simulink model "Solar_PV_IV_PV_Characteristics"  (R2024b)
settings: Solver=VariableStepAuto  StartTime=0.0  StopTime=4  RelTol=1e-3
values from neighbouring files (symbols this model uses):
  Ego = 1.1    [Soalr_Modeling_Parameters.m]
  Isc = 7.95    [Soalr_Modeling_Parameters.m]
  k = 1.380648e-23    [Soalr_Modeling_Parameters.m]
  ki = 0.0032    [Soalr_Modeling_Parameters.m]
  n = 1.29    [Soalr_Modeling_Parameters.m]
  Ns = 60    [Soalr_Modeling_Parameters.m]
  q = 1.602e-19    [Soalr_Modeling_Parameters.m]
  Rs = 0.1896    [Soalr_Modeling_Parameters.m]
  Rsh = 106.18    [Soalr_Modeling_Parameters.m]
  Tn = 298    [Soalr_Modeling_Parameters.m]
  Voc = 36.06    [Soalr_Modeling_Parameters.m]
libraries: simulink x1
settings Model: Creator=MULUK  LastModifiedBy=MULUK

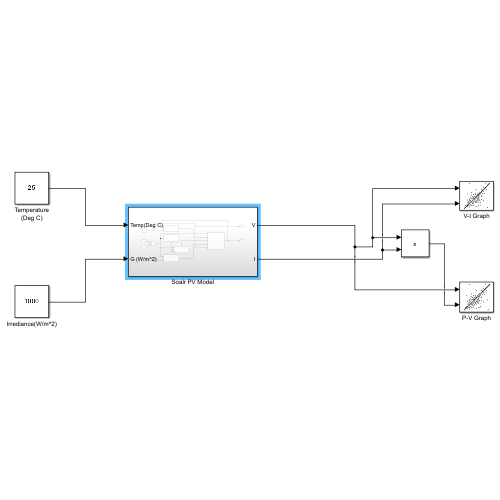
[thumbnail: Simulink's stored preview of the top-level diagram]
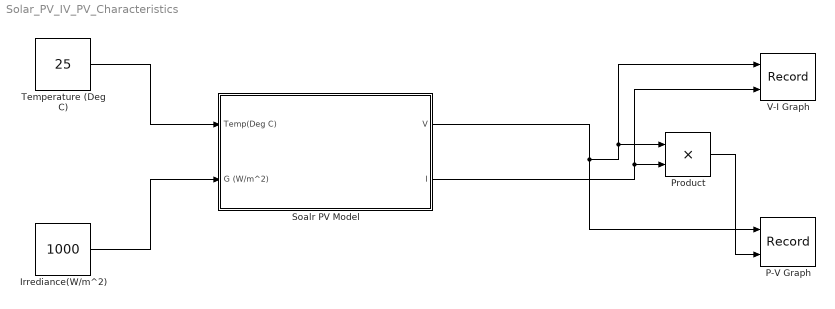
== system Solar_PV_IV_PV_Characteristics ==
  Irrediance(W/m^2) : Constant  Value=1000
  P-V Graph : Record  FileSettingsInternal="{\"entries\":[{\"content\":{\"excelSettings\":{\"content\":{},\"type\":\"Streamout.ExcelSettings\"}},\"type\":\"Streamout.FileSettingStorage\",\"uuid\":\"\"}],\"packageUris\":[\"http:\\/\\/schema.mathworks.com\\/mf0\\/streamout_blocks\\/R2020a\"],\"version\":\"1.0\"}"  Layout=[1 1]  SignalsInternal="{\"entries\":[{\"content\":{\"signals\":[{\"content\":{\"blockPath\":[],\"dimensions\":[1],\"domain\":\"\",\"lineColor\":\"#a2142f\",\"plots\":[ 1 ],\"port\":1,\"sid\":[\"\"],\"signalID\":1,\"signalName\":\"Soalr PV Model:1\"},\"type\":\"RecordBlkView.Signal\",\"uuid\":\"\"},{\"content\":{\"blockPath\":[],\"dimensions\":[1],\"domain\":\"\",\"lineColor\":\"#139fff\",\"plots\":[ 1 ],\"port\":2,\"sid\":[\"\"],\"signalID\":2,\"signalName\":\"Product\"},\"type\":\"RecordBlkView.Signal\",\"uuid\":\"\"}]},\"type\":\"RecordBlkView.InputSignals\",\"uuid\":\"\"}],\"packageUris\":[\"http:\\/\\/schema.mathworks.com\\/mf0\\/streamout_blocks\\/R2020a\"],\"version\":\"1.0\"}"  VisualizationBindings="{\"xyplotplugin\":{\"info\":[{\"series\":[{\"bindingParametersList\":[{\"parameter\":\"X-Axis\",\"signalID\":1,\"signalName\":\"Soalr PV Model:1\"},{\"parameter\":\"Y-Axis\",\"signalID\":2,\"signalName\":\"Product\"}],\"seriesID\":0}],\"subplotID\":1}]}}"  CompatibilityTag=XY
  Product : Product
  Soalr PV Model : Subsystem
  Temperature (Deg C) : Constant  Value=25
  V-I Graph : Record  FileSettingsInternal="{\"entries\":[{\"content\":{\"excelSettings\":{\"content\":{},\"type\":\"Streamout.ExcelSettings\"}},\"type\":\"Streamout.FileSettingStorage\",\"uuid\":\"\"}],\"packageUris\":[\"http:\\/\\/schema.mathworks.com\\/mf0\\/streamout_blocks\\/R2020a\"],\"version\":\"1.0\"}"  Layout=[1 1]  SignalsInternal="{\"entries\":[{\"content\":{\"signals\":[{\"content\":{\"blockPath\":[],\"dimensions\":[1],\"domain\":\"\",\"lineColor\":\"#a2142f\",\"plots\":[ 1 ],\"port\":1,\"sid\":[\"\"],\"signalID\":1,\"signalName\":\"Soalr PV Model:1\"},\"type\":\"RecordBlkView.Signal\",\"uuid\":\"\"},{\"content\":{\"blockPath\":[],\"dimensions\":[1],\"domain\":\"\",\"lineColor\":\"#139fff\",\"plots\":[ 1 ],\"port\":2,\"sid\":[\"\"],\"signalID\":2,\"signalName\":\"Soalr PV Model:2\"},\"type\":\"RecordBlkView.Signal\",\"uuid\":\"\"}]},\"type\":\"RecordBlkView.InputSignals\",\"uuid\":\"\"}],\"packageUris\":[\"http:\\/\\/schema.mathworks.com\\/mf0\\/streamout_blocks\\/R2020a\"],\"version\":\"1.0\"}"  VisualizationBindings="{\"xyplotplugin\":{\"info\":[{\"series\":[{\"bindingParametersList\":[{\"parameter\":\"X-Axis\",\"signalID\":1,\"signalName\":\"Soalr PV Model:1\"},{\"parameter\":\"Y-Axis\",\"signalID\":2,\"signalName\":\"Soalr PV Model:2\"}],\"seriesID\":0}],\"subplotID\":1}]}}"  CompatibilityTag=XY
  wires:
  Temperature (Deg C)/1 -> Soalr PV Model/1(Temp(Deg C))
  Irrediance(W/m^2)/1 -> Soalr PV Model/2(G (W/m^2))
  Soalr PV Model/1(V) -> P-V Graph/1, Product/1, V-I Graph/1
  Soalr PV Model/2(I) -> V-I Graph/2, Product/2
  Product/1 -> P-V Graph/2

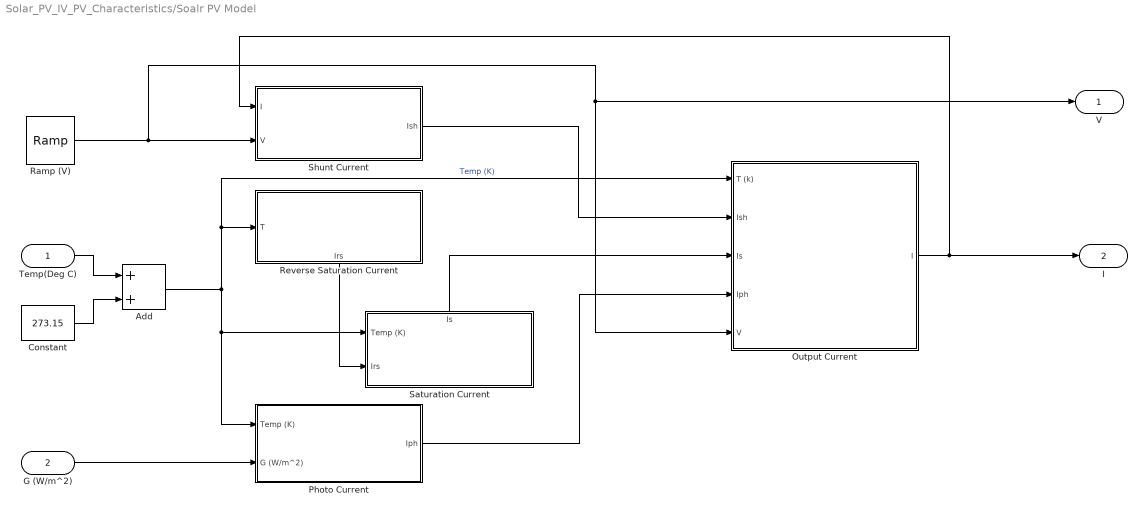
== system Solar_PV_IV_PV_Characteristics/Soalr PV Model ==
  Temp(Deg C) : Inport
  G (W/m^2) : Inport  Port=2
  " Saturation Current" : Subsystem
      settings: PortSchema="{\"entries\":[{\"content\":{\"sides\":[{\"content\":{\"connectorIds\":[\"In1\",\"In2\"]},\"type\":\"ConnectorPlacement.EquallySpacedRectSide\",\"uuid\":\"228251db-ac4b-41cf-ba5c-a510b5a8f8e4\"},{\"content\":{\"side\":\"RIGHT\"},\"type\":\"ConnectorPlacement.EquallySpacedRectSide\",\"uuid\":\"dc30eacc-74c4-4b6b-93d0-5a4bc4de7db7\"},{\"content\":{\"connectorIds\":[\"Out1\"],\"side\":\"TOP\"},\"type\":\"ConnectorPlacement.EquallySpacedRectSide\",\"uuid\":\"0f21fec9-16ef-4863-8682-a91fb4282025\"}]},\"type\":\"ConnectorPlacement.EquallySpacedConnector\",\"uuid\":\"707e5a0b-264d-4615-9fee-634224bb9e7b\"}],\"packageUris\":[\"http://schema.mathworks.com/mf0/Connector/R2020b\"],\"version\":\"1.0\"}"
  Add : Sum
  Constant : Constant  Value=273.15
  Output Current : Subsystem
  Photo Current : Subsystem
  Ramp (V) : simulink/Sources/Ramp  slope=10  start=0  InitialOutput=0
  Reverse Saturation Current : Subsystem
      settings: PortSchema="{\"entries\":[{\"content\":{\"sides\":[{\"content\":{\"connectorIds\":[\"In1\"]},\"type\":\"ConnectorPlacement.EquallySpacedRectSide\",\"uuid\":\"15512ed6-b5a7-405b-8341-08cd34b41276\"},{\"content\":{\"side\":\"RIGHT\"},\"type\":\"ConnectorPlacement.EquallySpacedRectSide\",\"uuid\":\"2cf76314-964e-48ba-8c80-893730139cda\"},{\"content\":{\"side\":\"TOP\"},\"type\":\"ConnectorPlacement.EquallySpacedRectSide\",\"uuid\":\"5ff35256-eb4a-4971-9008-324c8c50e0f9\"},{\"content\":{\"connectorIds\":[\"Out1\"],\"side\":\"BOTTOM\"},\"type\":\"ConnectorPlacement.EquallySpacedRectSide\",\"uuid\":\"1ee23ac2-1bc7-4858-ab4d-5fdcca5de137\"}]},\"type\":\"ConnectorPlacement.EquallySpacedConnector\",\"uuid\":\"a755481f-b56d-49f1-ba2a-78615b253991\"}],\"packageUris\":[\"http://schema.mathworks.com/mf0/Connector/R2020b\"],\"version\":\"1.0\"}"
  "Shunt Current " : Subsystem
  V : Outport
  I : Outport  Port=2
  wires:
  Temp(Deg C)/1 -> Add/1
  Constant/1 -> Add/2
  Add/1 -> Output Current/1(T (k)), Reverse Saturation Current/1(T), Photo Current/1(Temp (K)), " Saturation Current"/1(Temp (K))  "Temp (K)"
  G (W/m^2)/1 -> Photo Current/2(G (W/m^2))
  Reverse Saturation Current/1(Irs) -> " Saturation Current"/2(Irs)
  "Shunt Current "/1(Ish) -> Output Current/2(Ish)
  Photo Current/1(Iph) -> Output Current/4(Iph)
  " Saturation Current"/1(Is) -> Output Current/3(Is)
  Output Current/1(I) -> I/1, "Shunt Current "/1(I)
  Ramp (V)/1 -> V/1, Output Current/5(V), "Shunt Current "/2(V)

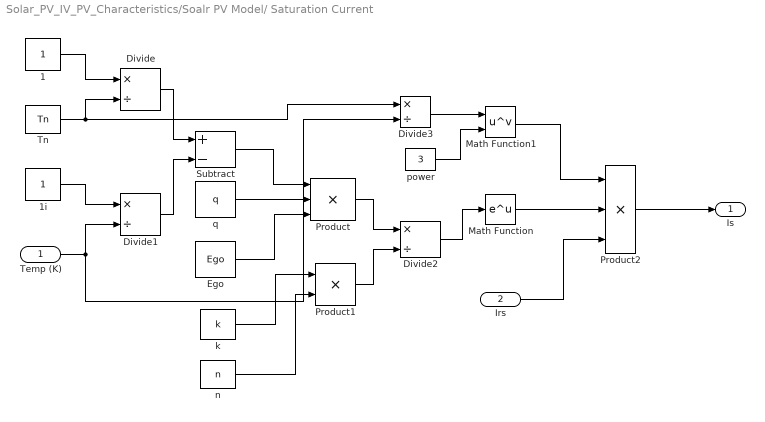
== system Solar_PV_IV_PV_Characteristics/Soalr PV Model/ Saturation Current ==
  Temp (K) : Inport
  Irs : Inport  Port=2
  1 : Constant
  1i : Constant
  Divide{,1..3} (4 alike) : Product  Inputs=*/
  Ego : Constant  Value=Ego
  Math Function : Math
  Math Function1 : Math  Operator=pow
  Product : Product  Inputs=3
  Product1 : Product
  Product2 : Product  Inputs=3
  Subtract : Sum  Inputs=+-
  Tn : Constant  Value=Tn
  k : Constant  Value=k
  n : Constant  Value=n
  power : Constant  Value=3
  q : Constant  Value=q
  Is : Outport
  wires:
  1/1 -> Divide/1
  Tn/1 -> Divide/2, Divide3/1
  1i/1 -> Divide1/1
  Temp (K)/1 -> Divide1/2, Divide3/2
  Divide/1 -> Subtract/1
  Divide1/1 -> Subtract/2
  Subtract/1 -> Product/1
  q/1 -> Product/2
  Ego/1 -> Product/3
  k/1 -> Product1/1
  n/1 -> Product1/2
  Product/1 -> Divide2/1
  Product1/1 -> Divide2/2
  Divide2/1 -> Math Function/1
  Divide3/1 -> Math Function1/1
  power/1 -> Math Function1/2
  Math Function/1 -> Product2/2
  Math Function1/1 -> Product2/1
  Irs/1 -> Product2/3
  Product2/1 -> Is/1

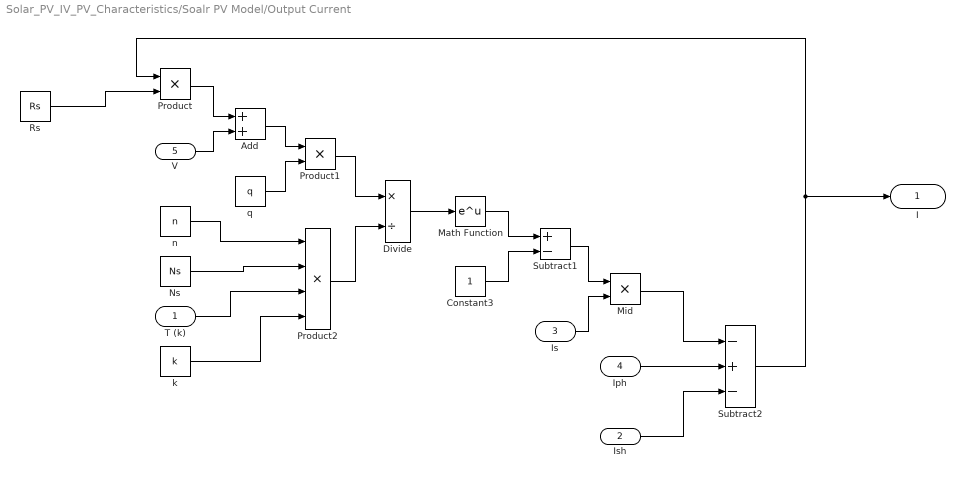
== system Solar_PV_IV_PV_Characteristics/Soalr PV Model/Output Current ==
  T (k) : Inport
  Ish : Inport  Port=2
  Is : Inport  Port=3
  Iph : Inport  Port=4
  V : Inport  Port=5
  Add : Sum
  Constant3 : Constant
  Divide : Product  Inputs=*/
  Math Function : Math
  Mid : Product
  Ns : Constant  Value=Ns
  Product : Product
  Product1 : Product
  Product2 : Product  Inputs=4
  Rs : Constant  Value=Rs
  Subtract1 : Sum  Inputs=+-
  Subtract2 : Sum  Inputs=-+-
  k : Constant  Value=k
  n : Constant  Value=n
  q : Constant  Value=q
  I : Outport
  wires:
  Subtract2/1 -> Product/1, I/1
  Rs/1 -> Product/2
  Product/1 -> Add/1
  V/1 -> Add/2
  q/1 -> Product1/2
  Add/1 -> Product1/1
  n/1 -> Product2/1
  T (k)/1 -> Product2/3
  k/1 -> Product2/4
  Ns/1 -> Product2/2
  Product1/1 -> Divide/1
  Product2/1 -> Divide/2
  Divide/1 -> Math Function/1
  Math Function/1 -> Subtract1/1
  Constant3/1 -> Subtract1/2
  Subtract1/1 -> Mid/1
  Is/1 -> Mid/2
  Mid/1 -> Subtract2/1
  Iph/1 -> Subtract2/2
  Ish/1 -> Subtract2/3

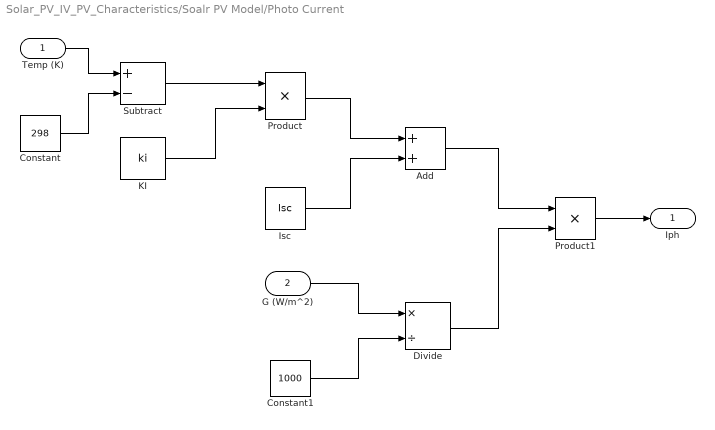
== system Solar_PV_IV_PV_Characteristics/Soalr PV Model/Photo Current ==
  Temp (K) : Inport
  G (W/m^2) : Inport  Port=2
  Add : Sum
  Constant : Constant  Value=298
  Constant1 : Constant  Value=1000
  Divide : Product  Inputs=*/
  Isc : Constant  Value=Isc
  KI : Constant  Value=ki
  Product : Product
  Product1 : Product
  Subtract : Sum  Inputs=+-
  Iph : Outport
  wires:
  Temp (K)/1 -> Subtract/1
  Constant/1 -> Subtract/2
  Subtract/1 -> Product/1
  KI/1 -> Product/2
  Product/1 -> Add/1
  Isc/1 -> Add/2
  G (W/m^2)/1 -> Divide/1
  Constant1/1 -> Divide/2
  Add/1 -> Product1/1
  Divide/1 -> Product1/2
  Product1/1 -> Iph/1

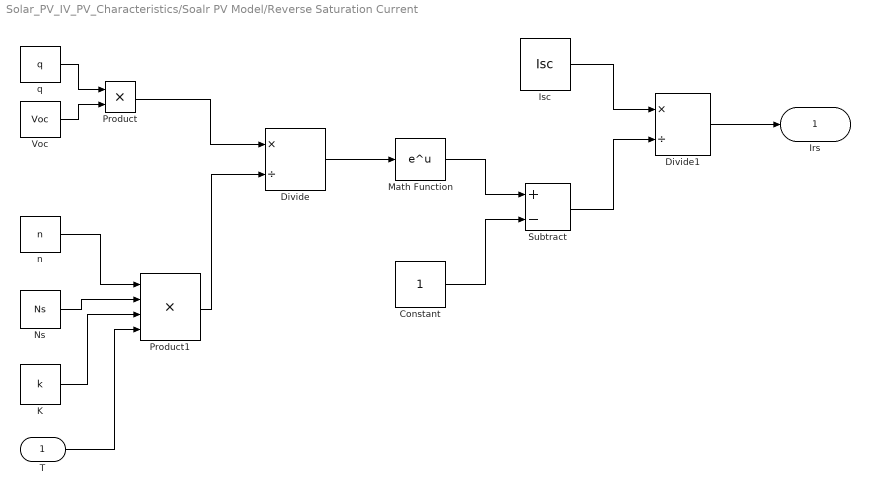
== system Solar_PV_IV_PV_Characteristics/Soalr PV Model/Reverse Saturation Current ==
  T : Inport
  Constant : Constant
  Divide : Product  Inputs=*/
  Divide1 : Product  Inputs=*/
  Isc : Constant  Value=Isc
  K : Constant  Value=k
  Math Function : Math
  Ns : Constant  Value=Ns
  Product : Product
  Product1 : Product  Inputs=4
  Subtract : Sum  Inputs=+-
  Voc : Constant  Value=Voc
  n : Constant  Value=n
  q : Constant  Value=q
  Irs : Outport
  wires:
  q/1 -> Product/1
  Voc/1 -> Product/2
  n/1 -> Product1/1
  Ns/1 -> Product1/2
  K/1 -> Product1/3
  T/1 -> Product1/4
  Product/1 -> Divide/1
  Product1/1 -> Divide/2
  Divide/1 -> Math Function/1
  Math Function/1 -> Subtract/1
  Constant/1 -> Subtract/2
  Isc/1 -> Divide1/1
  Subtract/1 -> Divide1/2
  Divide1/1 -> Irs/1

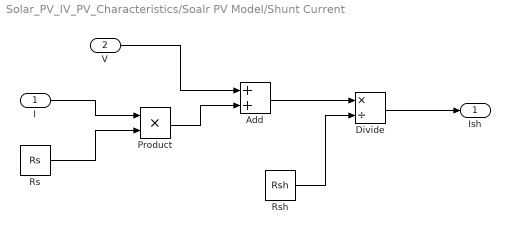
== system Solar_PV_IV_PV_Characteristics/Soalr PV Model/Shunt Current  ==
  I : Inport
  V : Inport  Port=2
  Add : Sum
  Divide : Product  Inputs=*/
  Product : Product
  Rs : Constant  Value=Rs
  Rsh : Constant  Value=Rsh
  Ish : Outport
  wires:
  I/1 -> Product/1
  Rs/1 -> Product/2
  Product/1 -> Add/2
  V/1 -> Add/1
  Add/1 -> Divide/1
  Rsh/1 -> Divide/2
  Divide/1 -> Ish/1
